simulink model "SimulationLoop_Cpp"  (R2025b)
settings: Solver=VariableStepAuto  StartTime=0.0  StopTime=50  RelTol=1e-3
InitFcn:
  | clear cpp_controller_mex_wrap
values from neighbouring files (symbols this model uses):
  Checkpoints = 0.0 0.0 0.0 0.0 0.0 3.0 0.0 3.0 3.0 3.0 3.0 3.0 3.0 0.0 3.0 0.0 0.0 3.0 0.0 0.0 0.0 0.0 0.0 0.0    [Variables.sldd]
  constantsASTRA = constructConstants    [LoadSimulation.m]    (also in Variables.sldd = 1.275
                0.5
                9.80145
          ; test.m = getEntry(dataSect, 'constantsASTRA'))
  distMode = 1.0    [Variables.sldd]
  dt = 0.005    [Variables.sldd]
  dt_SIM = 0.001    [Variables.sldd]
  HoldTimeReqs = 7.0 5.0 3.0 3.0 3.0 3.0 0.0 0.2    [Variables.sldd]
  IMU_Rate = 1000.0    [Variables.sldd]
  magDistMatrix = 1.0107533427909221 0.036677700291901733 -0.04517693722007296 0.01724346640736241 1.0063753047971795 -0.026153765926105469 -0.0086718404461136721 0.0068524893307729982 1.0715679387945152    [Variables.sldd]
  q = x(7:9)    [TEST1.m]
  u0 = [0; 0; constantsASTRA.g * constantsASTRA.m; 0]    [LoadSimulation.m]    (also in Variables.sldd = 0.0 0.0 12.49684875 0.0)
  x0 = zeros(18,1)    [LoadSimulation.m]    (also in Variables.sldd = 1.0 0.0 0.0 0.0 0.0 0.0 0.0 0.0 0.0 0.0 0.0 0.0 0.0 0.0 0.0 ; run_sim.m = zeros(12,1))
undefined symbols (not defined in the file or in its folder): DiscIntNeverNeededParam, F, Light, MIL
libraries: aerolibnav x2, aerolibwind2 x1, simulink x1
settings Model: PacingRate=5  Creator=antho  LastModifiedBy=pplat
settings OptimizationCC: AccelVerboseBuild=on

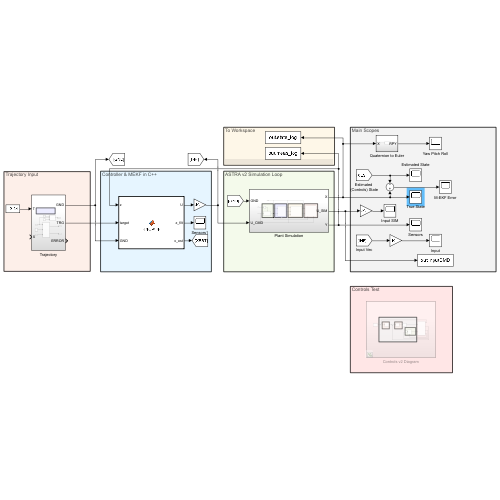
[thumbnail: Simulink's stored preview of the top-level diagram]
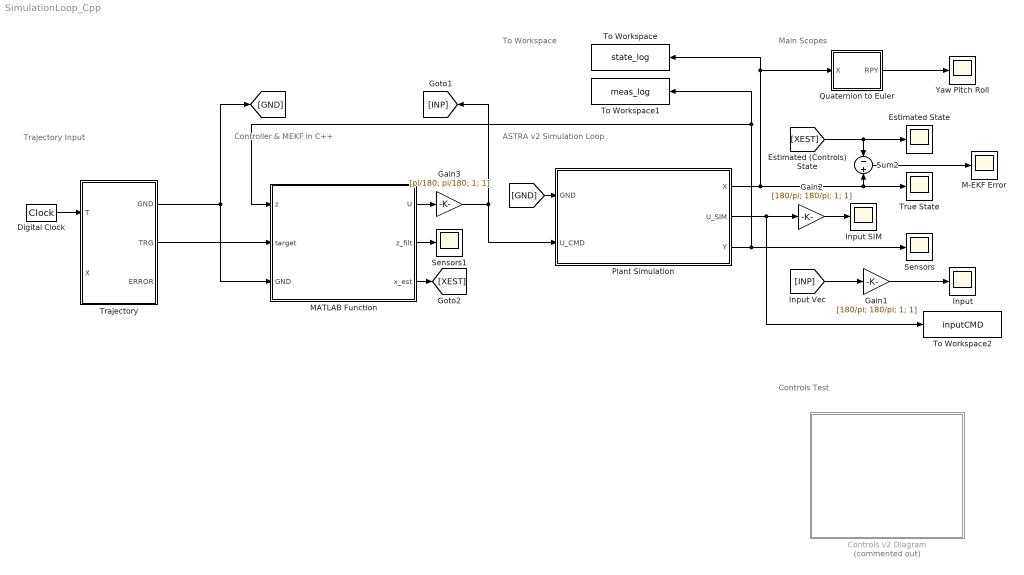
== system SimulationLoop_Cpp ==
  note: To Workspace
  note: Controls Test
  note: Main Scopes
  note: Trajectory Input
  note: Controller & MEKF in C++
  note: ASTRA v2 Simulation Loop
  Controls v2 Diagram : Subsystem  Commented=on
  Digital Clock : DigitalClock  SampleTime=dt_SIM
  Estimated State : Scope
      settings: ActiveDisplayYMinimum=-0.606468253752392  ActiveDisplayYMaximum=3.4359511007845942
  Gain1 : Gain  Gain=[180/pi; 180/pi; 1; 1]
  Gain2 : Gain  Gain=[180/pi; 180/pi; 1; 1]
  Gain3 : Gain  Gain=[pi/180; pi/180; 1; 1]
  Input : Scope
      settings: ActiveDisplayYMinimum=-13.087499976158142  ActiveDisplayYMaximum=17.787499785423279  DataLoggingVariableName=ScopeData6
  Input SIM : Scope
      settings: ActiveDisplayYMinimum=-9.3285969360922252  ActiveDisplayYMaximum=17.369726851522856  DataLoggingVariableName=ScopeData4
  M-EKF Error : Scope
      settings: ActiveDisplayYMinimum=-0.067271632908363993  ActiveDisplayYMaximum=0.0634163897991504  DataLoggingVariableName=ScopeData2
  MATLAB Function : MATLAB Function  TreatAsAtomicUnit=on
  Plant Simulation : Subsystem
  Quaternion to Euler : Subsystem
  Sensors : Scope
      settings: ActiveDisplayYMinimum=-2.5158529896476529  ActiveDisplayYMaximum=2.4618166614919  DataLoggingVariableName=ScopeData3
  Sensors1 : Scope
      settings: ActiveDisplayYMinimum=-5.9307053983211508  ActiveDisplayYMaximum=34.316149324178696  DataLoggingVariableName=ScopeData9
  Sum2 : Sum  Inputs=-|+
  To Workspace : ToWorkspace  VariableName=state_log  SaveFormat=Timeseries  SampleTime=-1
  To Workspace1 : ToWorkspace  VariableName=meas_log  SaveFormat=Timeseries  SampleTime=-1
  To Workspace2 : ToWorkspace  VariableName=inputCMD  SaveFormat=Timeseries  SampleTime=-1
  Trajectory : Subsystem
  True State : Scope
      settings: ActiveDisplayYMinimum=-0.46402431479384865  ActiveDisplayYMaximum=3.346767927011304
  Yaw Pitch Roll : Scope
      settings: ActiveDisplayYMinimum=-2.3625770420783638  ActiveDisplayYMaximum=6.5496164506169734  DataLoggingVariableName=ScopeData7
  wires:
  Digital Clock/1 -> Trajectory/1(T)
  [XEST] -> Sum2/1, Estimated State/1
  Sum2/1 -> M-EKF Error/1
  MATLAB Function/1(U) -> Gain3/1
  Trajectory/1(GND) -> MATLAB Function/3(GND), [GND]
  [INP] -> Gain1/1
  Gain1/1 -> Input/1
  Gain2/1 -> Input SIM/1
  Plant Simulation/2(U_SIM) -> To Workspace2/1, Gain2/1
  Quaternion to Euler/1(RPY) -> Yaw Pitch Roll/1
  [GND] -> Plant Simulation/1(GND)
  Plant Simulation/3(Y) -> To Workspace1/1, MATLAB Function/1(z), Sensors/1
  Plant Simulation/1(X) -> Sum2/2, True State/1, Quaternion to Euler/1(X), To Workspace/1
  Trajectory/2(TRG) -> MATLAB Function/2(target)
  MATLAB Function/2(z_filt) -> Sensors1/1
  MATLAB Function/3(x_est) -> [XEST]
  Gain3/1 -> Plant Simulation/2(U_CMD), [INP]

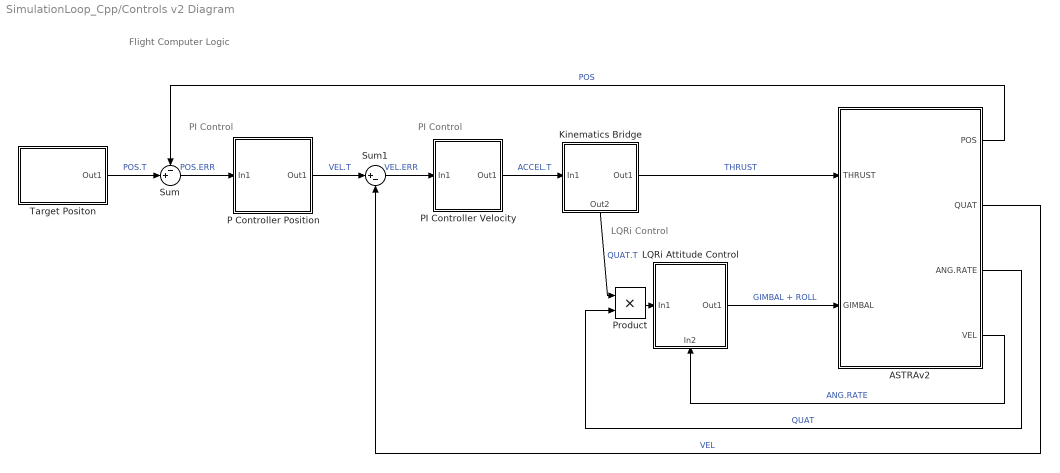
== system SimulationLoop_Cpp/Controls v2 Diagram ==
  note: PI Control
  note: Flight Computer Logic
  note: PI Control
  note: LQRi Control
  ASTRAv2 : Subsystem
  Kinematics Bridge : Subsystem
      settings: PortSchema="{\"entries\":[{\"content\":{\"sides\":[{\"content\":{\"connectorIds\":[\"In1\"]},\"type\":\"ConnectorPlacement.EquallySpacedRectSide\",\"uuid\":\"14f1819f-c5b0-4857-8a3f-059930327852\"},{\"content\":{\"connectorIds\":[\"Out1\"],\"side\":\"RIGHT\"},\"type\":\"ConnectorPlacement.EquallySpacedRectSide\",\"uuid\":\"f1c93ae3-8d17-4b74-967d-9d6328e115fb\"},{\"content\":{\"side\":\"TOP\"},\"type\":\"ConnectorPlacement.EquallySpacedRectSide\",\"uuid\":\"bc82f49d-1f27-4136-b175-63a6ad0dbf5b\"},{\"content\":{\"connectorIds\":[\"Out2\"],\"side\":\"BOTTOM\"},\"type\":\"ConnectorPlacement.EquallySpacedRectSide\",\"uuid\":\"6dcf9527-a6d9-4dea-a2bb-d98c67e6f046\"}]},\"type\":\"ConnectorPlacement.EquallySpacedConnector\",\"uuid\":\"f166f20b-cbf6-467f-83b3-19efe4727134\"}],\"packageUris\":[\"http://schema.mathworks.com/mf0/Connector/R2020b\"],\"version\":\"1.0\"}"
  LQRi Attitude Control : Subsystem
      settings: PortSchema="{\"entries\":[{\"content\":{\"sides\":[{\"content\":{\"connectorIds\":[\"In1\"]},\"type\":\"ConnectorPlacement.EquallySpacedRectSide\",\"uuid\":\"cd9cee5f-4e02-4c25-b158-b6d381dcbc8d\"},{\"content\":{\"connectorIds\":[\"Out1\"],\"side\":\"RIGHT\"},\"type\":\"ConnectorPlacement.EquallySpacedRectSide\",\"uuid\":\"2ef087dd-7fcc-4555-b2da-05ccf598bd0a\"},{\"content\":{\"side\":\"TOP\"},\"type\":\"ConnectorPlacement.EquallySpacedRectSide\",\"uuid\":\"5427ed8c-500e-4860-8e5f-93d13574dd24\"},{\"content\":{\"connectorIds\":[\"In2\"],\"side\":\"BOTTOM\"},\"type\":\"ConnectorPlacement.EquallySpacedRectSide\",\"uuid\":\"f48b80df-9658-4fd9-b967-6adbaff8a875\"}]},\"type\":\"ConnectorPlacement.EquallySpacedConnector\",\"uuid\":\"547d8ec4-1c4e-4f3b-85b8-72bd650a229d\"}],\"packageUris\":[\"http://schema.mathworks.com/mf0/Connector/R2020b\"],\"version\":\"1.0\"}"
  P Controller Position : Subsystem
  PI Controller Velocity : Subsystem
  Product : Product
  Sum : Sum  Inputs=-+|
  Sum1 : Sum  Inputs=|+-
  Target Positon : Subsystem
  wires:
  P Controller Position/1(Out1) -> Sum1/1  "VEL.T"
  Sum1/1 -> PI Controller Velocity/1(In1)  "VEL.ERR"
  PI Controller Velocity/1(Out1) -> Kinematics Bridge/1(In1)  "ACCEL.T"
  Sum/1 -> P Controller Position/1(In1)  "POS.ERR"
  Kinematics Bridge/2(Out2) -> Product/1  "QUAT.T"
  Product/1 -> LQRi Attitude Control/1(In1)
  LQRi Attitude Control/1(Out1) -> ASTRAv2/2("GIMBAL ")  "GIMBAL + ROLL"
  Kinematics Bridge/1(Out1) -> ASTRAv2/1(THRUST)  "THRUST"
  Target Positon/1(Out1) -> Sum/2  "POS.T"
  ASTRAv2/1(POS) -> Sum/1  "POS"
  ASTRAv2/2(QUAT) -> Sum1/2  "VEL"
  ASTRAv2/3(ANG.RATE) -> Product/2  "QUAT"
  ASTRAv2/4(VEL) -> LQRi Attitude Control/2(In2)  "ANG.RATE"

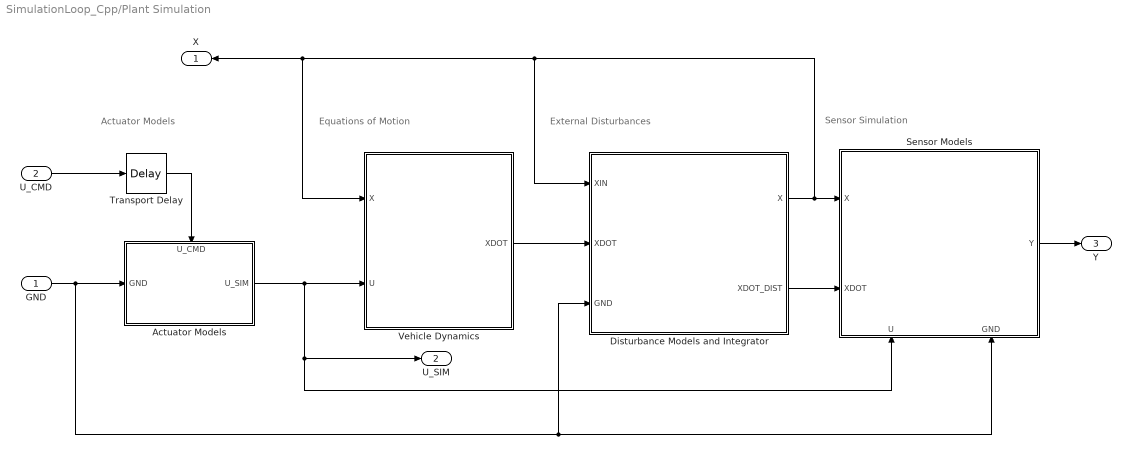
== system SimulationLoop_Cpp/Plant Simulation ==
  note: Equations of Motion
  note: Actuator Models
  note: External Disturbances
  note: Sensor Simulation
  GND : Inport
  U_CMD : Inport  Port=2
  Actuator Models : Subsystem
      settings: PortSchema="{\"entries\":[{\"content\":{\"sides\":[{\"content\":{\"connectorIds\":[\"In1\"]},\"type\":\"ConnectorPlacement.EquallySpacedRectSide\",\"uuid\":\"54343072-6023-41e9-a0f6-81f6bed17e05\"},{\"content\":{\"connectorIds\":[\"Out1\"],\"side\":\"RIGHT\"},\"type\":\"ConnectorPlacement.EquallySpacedRectSide\",\"uuid\":\"2ed3290f-d38b-41d8-95ae-d88068502334\"},{\"content\":{\"connectorIds\":[\"In2\"],\"side\":\"TOP\"},\"type\":\"ConnectorPlacement.EquallySpacedRectSide\",\"uuid\":\"e9e41c57-b871-4be2-92e8-dfbbf995d6b0\"}]},\"type\":\"ConnectorPlacement.EquallySpacedConnector\",\"uuid\":\"c037521e-b20b-40c6-bb74-3aafe8fc1476\"}],\"packageUris\":[\"http://schema.mathworks.com/mf0/Connector/R2020b\"],\"version\":\"1.0\"}"
  Disturbance Models and Integrator : Subsystem
  Sensor Models : Subsystem
      settings: PortSchema="{\"entries\":[{\"content\":{\"sides\":[{\"content\":{\"connectorIds\":[\"In1\",\"In2\"]},\"type\":\"ConnectorPlacement.EquallySpacedRectSide\",\"uuid\":\"9bc4a206-bba4-4c50-88a9-89b0392ab722\"},{\"content\":{\"connectorIds\":[\"Out1\"],\"side\":\"RIGHT\"},\"type\":\"ConnectorPlacement.EquallySpacedRectSide\",\"uuid\":\"162bbd17-e1b8-4f29-9191-53e17e38d79d\"},{\"content\":{\"side\":\"TOP\"},\"type\":\"ConnectorPlacement.EquallySpacedRectSide\",\"uuid\":\"c56a23db-6a5c-435f-99fd-d50fc9dbdc94\"},{\"content\":{\"connectorIds\":[\"In3\",\"In4\"],\"side\":\"BOTTOM\"},\"type\":\"ConnectorPlacement.EquallySpacedRectSide\",\"uuid\":\"e0c2a0dc-3b7a-40ac-8345-28e7bf7b9405\"}]},\"type\":\"ConnectorPlacement.EquallySpacedConnector\",\"uuid\":\"d1c29f55-9be5-4f45-9d70-06beba2c2f44\"}],\"packageUris\":[\"http://schema.mathworks.com/mf0/Connector/R2020b\"],\"version\":\"1.0\"}"
  Transport Delay : TransportDelay  DelayTime=0.02  InitialOutput=u0
  Vehicle Dynamics : Subsystem
  X : Outport
  U_SIM : Outport  Port=2
  Y : Outport  Port=3
  wires:
  Vehicle Dynamics/1(XDOT) -> Disturbance Models and Integrator/2(XDOT)
  Sensor Models/1(Y) -> Y/1
  GND/1 -> Actuator Models/1(GND), Sensor Models/4(GND), Disturbance Models and Integrator/3(GND)
  Disturbance Models and Integrator/1(X) -> Disturbance Models and Integrator/1(XIN), Vehicle Dynamics/1(X), X/1, Sensor Models/1(X)
  Disturbance Models and Integrator/2(XDOT_DIST) -> Sensor Models/2(XDOT)
  Actuator Models/1(U_SIM) -> U_SIM/1, Sensor Models/3(U), Vehicle Dynamics/2(U)
  U_CMD/1 -> Transport Delay/1
  Transport Delay/1 -> Actuator Models/2(U_CMD)

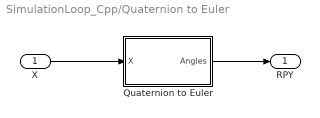
== system SimulationLoop_Cpp/Quaternion to Euler ==
  X : Inport
  Quaternion to Euler : MATLAB Function  TreatAsAtomicUnit=on
  RPY : Outport
  wires:
  X/1 -> Quaternion to Euler/1(X)
  Quaternion to Euler/1(Angles) -> RPY/1

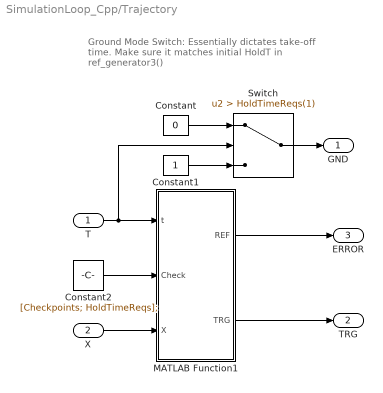
== system SimulationLoop_Cpp/Trajectory ==
  note: Ground Mode Switch:
      | Essentially dictates take-off time.
      | Make sure it matches initial HoldT
      | in ref_generator3()
  T : Inport
  X : Inport  Port=2
  Constant : Constant  Value=0
  Constant1 : Constant
  Constant2 : Constant  Value=[Checkpoints; HoldTimeReqs];
  MATLAB Function1 : MATLAB Function  TreatAsAtomicUnit=on
  Switch : Switch  Criteria=u2 > Threshold  Threshold=HoldTimeReqs(1)  SaturateOnIntegerOverflow=off  InputSameDT=off
  GND : Outport
  TRG : Outport  Port=2
  ERROR : Outport  Port=3
  wires:
  T/1 -> Switch/2, MATLAB Function1/1(t)
  X/1 -> MATLAB Function1/3(X)
  MATLAB Function1/1(REF) -> ERROR/1
  Constant/1 -> Switch/1
  Constant1/1 -> Switch/3
  Switch/1 -> GND/1
  Constant2/1 -> MATLAB Function1/2(Check)
  MATLAB Function1/2(TRG) -> TRG/1

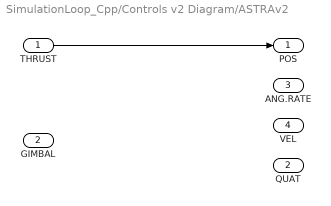
== system SimulationLoop_Cpp/Controls v2 Diagram/ASTRAv2 ==
  THRUST : Inport
  "GIMBAL " : Inport  Port=2
  POS : Outport
  QUAT : Outport  Port=2
  ANG.RATE : Outport  Port=3
  VEL : Outport  Port=4
  wires:
  THRUST/1 -> POS/1

== system SimulationLoop_Cpp/Controls v2 Diagram/Kinematics Bridge ==
  In1 : Inport
  Out1 : Outport
  Out2 : Outport  Port=2
  wires:
  In1/1 -> Out2/1, Out1/1

== system SimulationLoop_Cpp/Controls v2 Diagram/LQRi Attitude Control ==
  In1 : Inport
  In2 : Inport  Port=2
  Out1 : Outport
  wires:
  In1/1 -> Out1/1

== system SimulationLoop_Cpp/Controls v2 Diagram/P Controller Position ==
  In1 : Inport
  Out1 : Outport
  wires:
  In1/1 -> Out1/1

== system SimulationLoop_Cpp/Controls v2 Diagram/PI Controller Velocity ==
  In1 : Inport
  Out1 : Outport
  wires:
  In1/1 -> Out1/1

== system SimulationLoop_Cpp/Controls v2 Diagram/Target Positon ==
  Out1 : Outport
  wires:
  ? -> Out1/1

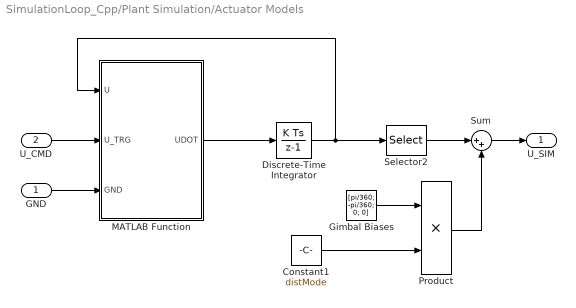
== system SimulationLoop_Cpp/Plant Simulation/Actuator Models ==
  GND : Inport
  U_CMD : Inport  Port=2
  Constant1 : Constant  Value=distMode
  Discrete-Time Integrator : DiscreteIntegrator  InitialCondition=[zeros(4,1); u0(3); 0]  SampleTime=-1  ICPrevOutput=DiscIntNeverNeededParam  ICPrevScaledInput=DiscIntNeverNeededParam
  Gimbal Biases : Constant  Value=[pi/360; -pi/360; 0; 0]
  MATLAB Function : MATLAB Function  TreatAsAtomicUnit=on
  Product : Product
  Selector2 : Selector  InputPortWidth=6  IndexOptions=Index vector (dialog)  Indices=[1 3 5 6]  OutputSizes=1
  Sum : Sum  Inputs=|++
  U_SIM : Outport
  wires:
  U_CMD/1 -> MATLAB Function/2(U_TRG)
  MATLAB Function/1(UDOT) -> Discrete-Time Integrator/1
  Discrete-Time Integrator/1 -> MATLAB Function/1(U), Selector2/1
  GND/1 -> MATLAB Function/3(GND)
  Sum/1 -> U_SIM/1
  Selector2/1 -> Sum/1
  Gimbal Biases/1 -> Product/1
  Product/1 -> Sum/2
  Constant1/1 -> Product/2

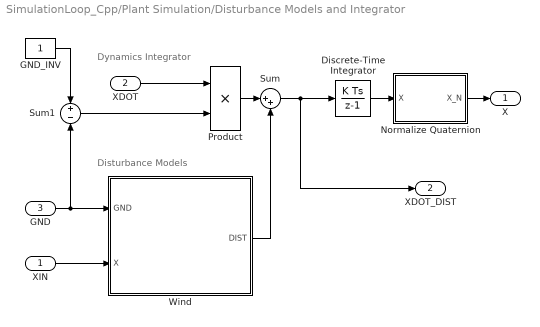
== system SimulationLoop_Cpp/Plant Simulation/Disturbance Models and Integrator ==
  note: Disturbance Models
  note: Dynamics Integrator
  XIN : Inport
  XDOT : Inport  Port=2
  GND : Inport  Port=3
  Discrete-Time Integrator : DiscreteIntegrator  InitialCondition=x0  SampleTime=-1  ICPrevOutput=DiscIntNeverNeededParam  ICPrevScaledInput=DiscIntNeverNeededParam
  GND_INV : Constant
  Normalize Quaternion : MATLAB Function  TreatAsAtomicUnit=on
  Product : Product
  Sum : Sum  Inputs=|++
  Sum1 : Sum  Inputs=+|-
  Wind : Subsystem
  X : Outport
  XDOT_DIST : Outport  Port=2
  wires:
  Discrete-Time Integrator/1 -> Normalize Quaternion/1(X)
  XIN/1 -> Wind/2(X)
  Wind/1(DIST) -> Sum/2
  XDOT/1 -> Product/1
  GND_INV/1 -> Sum1/1
  Sum1/1 -> Product/2
  GND/1 -> Wind/1(GND), Sum1/2
  Product/1 -> Sum/1
  Sum/1 -> Discrete-Time Integrator/1, XDOT_DIST/1
  Normalize Quaternion/1(X_N) -> X/1

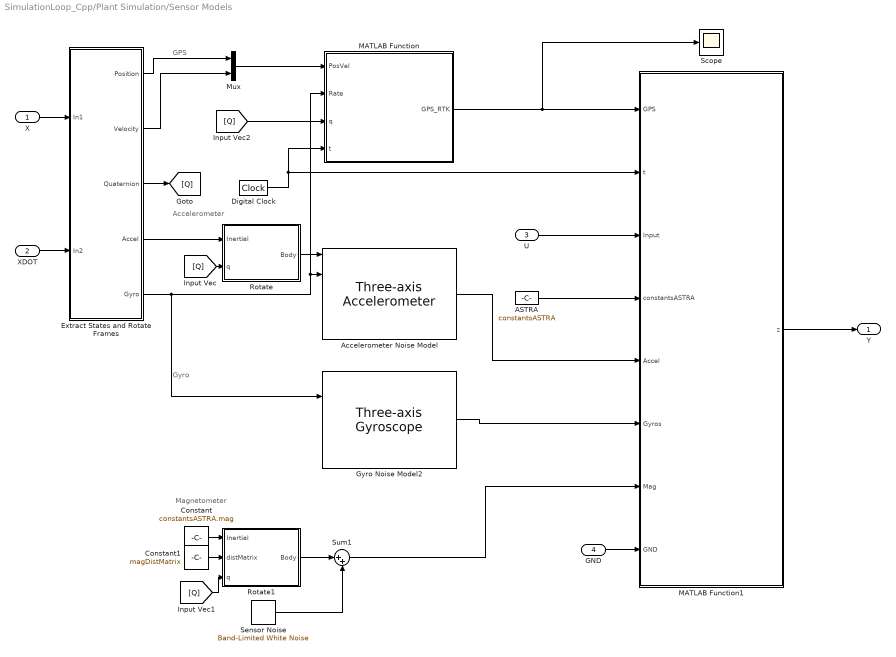
== system SimulationLoop_Cpp/Plant Simulation/Sensor Models ==
  note: Gyro
  note: Accelerometer
  note: Magnetometer
  note: GPS
  X : Inport
  XDOT : Inport  Port=2
  U : Inport  Port=3
  GND : Inport  Port=4
  ASTRA : Constant  Value=constantsASTRA  OutDataTypeStr=Bus: slBus1
  Accelerometer Noise Model : aerolibnav/Three-axis Accelerometer  units=Metric (MKS)  acc=[0 0 0.15]  gtype=on  dtype_a=on  w_a=190  z_a=0.707  a_sf_cc=eye(3)  a_bias=accelBias  a_Ts=1 / IMU_Rate  a_rand=on  a_seeds=[23093 23094 23095]  a_pow=ones(1,3) * 0.008^2 * 1 / IMU_Rate  a_sat="[-inf  -inf  -inf  inf inf inf]"
  Constant : Constant  Value=constantsASTRA.mag
  Constant1 : Constant  Value=magDistMatrix
  Digital Clock : DigitalClock  SampleTime=dt_SIM
  Extract States and Rotate Frames : Subsystem
  Gyro Noise Model2 : aerolibnav/Three-axis Gyroscope  dtype_g=on  w_g=190  z_g=0.707  g_sf_cc=eye(3)  g_bias=gyroBias  g_sen=0  g_Ts=1 / IMU_Rate  g_rand=on  g_seeds=[23093 23094 23095]  g_pow=ones(1,3) * 0.003^2 * dt  g_sat="[-inf  -inf  -inf  inf inf inf]"
  MATLAB Function : MATLAB Function  TreatAsAtomicUnit=on
  MATLAB Function1 : MATLAB Function  TreatAsAtomicUnit=on
  Mux : Mux  Inputs=2
  Rotate : MATLAB Function  TreatAsAtomicUnit=on
  Rotate1 : MATLAB Function  TreatAsAtomicUnit=on
  Scope : Scope
      settings: ActiveDisplayYMinimum=-1  ActiveDisplayYMaximum=1  DataLoggingVariableName=ScopeData10
  Sensor Noise : simulink/Sources/Band-Limited White Noise  Cov=(4E-4)^2  Ts=dt_SIM  seed=[23341,23342,23343]
  Sum1 : Sum  Inputs=|++
  Y : Outport
  wires:
  X/1 -> Extract States and Rotate Frames/1(In1)
  XDOT/1 -> Extract States and Rotate Frames/2(In2)
  Digital Clock/1 -> MATLAB Function/4(t), MATLAB Function1/2(t)
  Extract States and Rotate Frames/5(Gyro) -> Accelerometer Noise Model/2, MATLAB Function/2(Rate), Gyro Noise Model2/1
  Extract States and Rotate Frames/3(Quaternion) -> [Q]
  Rotate/1(Body) -> Accelerometer Noise Model/1
  Extract States and Rotate Frames/4(Accel) -> Rotate/1(Inertial)
  [Q] -> Rotate/2(q)
  Constant/1 -> Rotate1/1(Inertial)
  [Q] -> Rotate1/3(q)
  Sensor Noise/1 -> Sum1/2
  Rotate1/1(Body) -> Sum1/1
  Sum1/1 -> MATLAB Function1/7(Mag)
  MATLAB Function/1(GPS_RTK) -> Scope/1, MATLAB Function1/1(GPS)
  Accelerometer Noise Model/1 -> MATLAB Function1/5(Accel)
  Gyro Noise Model2/1 -> MATLAB Function1/6(Gyros)
  MATLAB Function1/1(z) -> Y/1
  ASTRA/1 -> MATLAB Function1/4(constantsASTRA)
  Extract States and Rotate Frames/2(Velocity) -> Mux/2
  Mux/1 -> MATLAB Function/1(PosVel)
  Extract States and Rotate Frames/1(Position) -> Mux/1
  U/1 -> MATLAB Function1/3(Input)
  GND/1 -> MATLAB Function1/8(GND)
  Constant1/1 -> Rotate1/2(distMatrix)
  [Q] -> MATLAB Function/3(q)

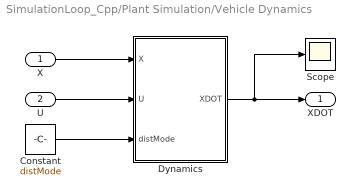
== system SimulationLoop_Cpp/Plant Simulation/Vehicle Dynamics ==
  X : Inport
  U : Inport  Port=2
  Constant : Constant  Value=distMode
  Dynamics : MATLAB Function  TreatAsAtomicUnit=on
  Scope : Scope
      settings: ActiveDisplayYMinimum=-0.093144832224715035  ActiveDisplayYMaximum=0.26958232579352592  DataLoggingVariableName=ScopeData11
  XDOT : Outport
  wires:
  Dynamics/1(XDOT) -> Scope/1, XDOT/1
  U/1 -> Dynamics/2(U)
  X/1 -> Dynamics/1(X)
  Constant/1 -> Dynamics/3(distMode)

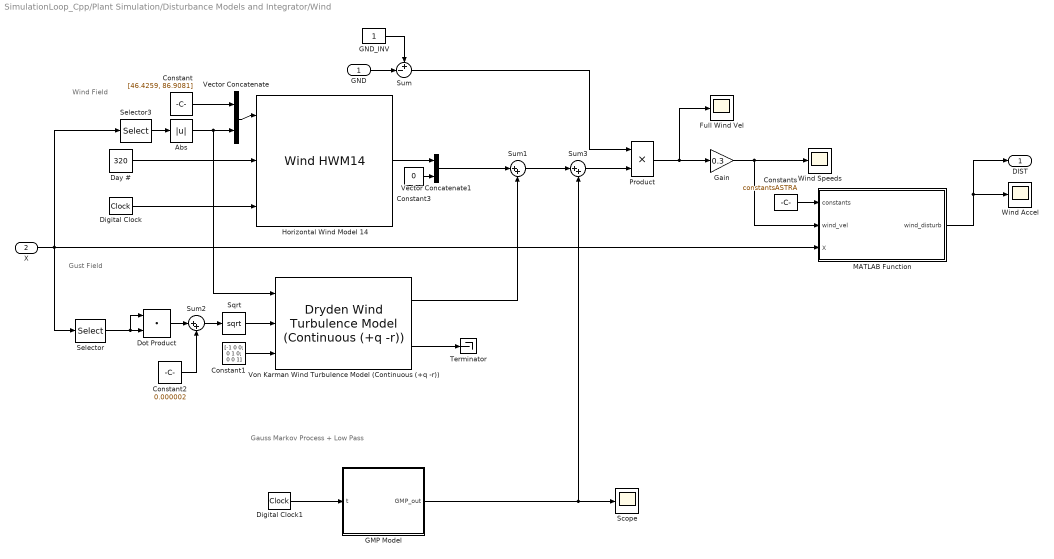
== system SimulationLoop_Cpp/Plant Simulation/Disturbance Models and Integrator/Wind ==
  note: Gauss Markov Process + Low Pass
  note: Gust Field
  note: Wind Field
  GND : Inport
  X : Inport  Port=2
  Abs : Abs  SaturateOnIntegerOverflow=off
  Constant : Constant  Value=[46.4259, 86.9081]
  Constant1 : Constant  Value=[-1 0 0; 0 1 0; 0 0 1]
  Constant2 : Constant  Value=0.000002
  Constant3 : Constant  Value=0
  Constants : Constant  Value=constantsASTRA  OutDataTypeStr=Bus: slBus1
  Day # : Constant  Value=320
  Digital Clock : DigitalClock  SampleTime=dt_SIM
  Digital Clock1 : DigitalClock  SampleTime=dt_SIM
  Dot Product : DotProduct  OutDataTypeStr=Inherit: Inherit via internal rule
  Full Wind Vel : Scope
      settings: ActiveDisplayYMinimum=-5.9330847029288414  ActiveDisplayYMaximum=4.4700897462030218  DataLoggingVariableName=ScopeData13
  GMP Model : MATLAB Function  TreatAsAtomicUnit=on
  GND_INV : Constant
  Gain : Gain  Gain=0.3
  Horizontal Wind Model 14 : WindHWM14
  MATLAB Function : MATLAB Function  TreatAsAtomicUnit=on
  Product : Product
  Scope : Scope
      settings: ActiveDisplayYMinimum=-2.8676060433464485  ActiveDisplayYMaximum=2.8612107779538238  DataLoggingVariableName=ScopeData14
  Selector : Selector  InputPortWidth=16  IndexOptions=Index vector (dialog)  Indices=[8:10]  OutputSizes=1
  Selector3 : Selector  InputPortWidth=16  IndexOptions=Index vector (dialog)  Indices=7  OutputSizes=1
  Sqrt : Sqrt
  Sum : Sum  Inputs=+-|
  Sum1 : Sum  Inputs=|++
  Sum2 : Sum  Inputs=|++
  Sum3 : Sum  Inputs=|++
  Terminator : Terminator
  Vector Concatenate : Concatenate
  Vector Concatenate1 : Concatenate
  Von Karman Wind Turbulence Model (Continuous (+q -r)) : aerolibwind2/Dryden Wind Turbulence Model  (Continuous (+q -r))  units=Metric (MKS)  spec=MIL-F-8785C  model=Continuous Von Karman (+q -r)  W20=15  Wdeg=0  TurbProb=10^-2 - Light  L_high=762  Wingspan=10  ts=0.1  Seed=[23341 23342 23343 23344]  T_on=on
      settings: LibrarySourceBlock=|
      | aerolibwind2/Von Karman Wind Turbulence Model
      | (Continuous (+q -r))
  Wind Accel : Scope
      settings: ActiveDisplayYMinimum=-0.93847040858698449  ActiveDisplayYMaximum=0.85102417935944119  DataLoggingVariableName=ScopeData5
  Wind Speeds : Scope
      settings: ActiveDisplayYMinimum=-6.0032131159962416  ActiveDisplayYMaximum=4.44789373969359  DataLoggingVariableName=ScopeData5
  DIST : Outport
  wires:
  Digital Clock/1 -> Horizontal Wind Model 14/3
  Day #/1 -> Horizontal Wind Model 14/2
  MATLAB Function/1(wind_disturb) -> DIST/1, Wind Accel/1
  Vector Concatenate/1 -> Horizontal Wind Model 14/1
  Selector3/1 -> Abs/1
  Constant/1 -> Vector Concatenate/1
  GND/1 -> Sum/2
  Sum/1 -> Product/1
  GND_INV/1 -> Sum/1
  Horizontal Wind Model 14/1 -> Vector Concatenate1/1
  Constants/1 -> MATLAB Function/1(constants)
  Selector/1 -> Dot Product/1, Dot Product/2
  Sqrt/1 -> Von Karman Wind Turbulence Model (Continuous (+q -r))/2
  Von Karman Wind Turbulence Model (Continuous (+q -r))/1 -> Sum1/2
  Constant1/1 -> Von Karman Wind Turbulence Model (Continuous (+q -r))/3
  Sum2/1 -> Sqrt/1
  Dot Product/1 -> Sum2/1
  Constant2/1 -> Sum2/2
  X/1 -> Selector3/1, MATLAB Function/3(X), Selector/1
  Abs/1 -> Vector Concatenate/2, Von Karman Wind Turbulence Model (Continuous (+q -r))/1
  Product/1 -> Full Wind Vel/1, Gain/1
  Vector Concatenate1/1 -> Sum1/1
  Constant3/1 -> Vector Concatenate1/2
  Von Karman Wind Turbulence Model (Continuous (+q -r))/2 -> Terminator/1
  Gain/1 -> Wind Speeds/1, MATLAB Function/2(wind_vel)
  Sum3/1 -> Product/2
  Sum1/1 -> Sum3/1
  GMP Model/1(GMP_out) -> Scope/1, Sum3/2
  Digital Clock1/1 -> GMP Model/1(t)

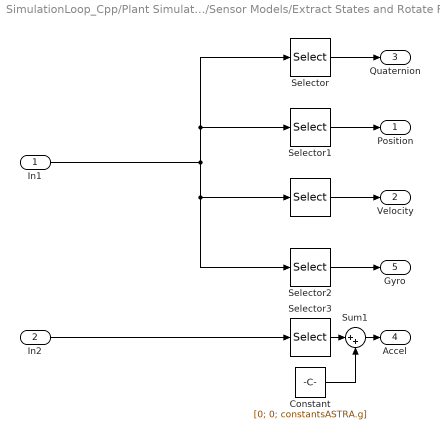
== system SimulationLoop_Cpp/Plant Simulation/Sensor Models/Extract States and Rotate Frames ==
  In1 : Inport
  In2 : Inport  Port=2
  "  " : Selector  InputPortWidth=16  IndexOptions=Index vector (dialog)  Indices=[8:10]  OutputSizes=1
  Constant : Constant  Value=[0; 0; constantsASTRA.g]
  Selector : Selector  InputPortWidth=16  IndexOptions=Index vector (dialog)  Indices=[1:4]  OutputSizes=1
  Selector1 : Selector  InputPortWidth=16  IndexOptions=Index vector (dialog)  Indices=[5:7]  OutputSizes=1
  Selector2 : Selector  InputPortWidth=16  IndexOptions=Index vector (dialog)  Indices=[11:13]  OutputSizes=1
  Selector3 : Selector  InputPortWidth=16  IndexOptions=Index vector (dialog)  Indices=[8:10]  OutputSizes=1
  Sum1 : Sum  Inputs=|++
  Position : Outport
  Velocity : Outport  Port=2
  Quaternion : Outport  Port=3
  Accel : Outport  Port=4
  Gyro : Outport  Port=5
  wires:
  Selector/1 -> Quaternion/1
  Selector1/1 -> Position/1
  "  "/1 -> Velocity/1
  Selector2/1 -> Gyro/1
  Selector3/1 -> Sum1/1
  Sum1/1 -> Accel/1
  Constant/1 -> Sum1/2
  In1/1 -> Selector1/1, Selector/1, Selector2/1, "  "/1
  In2/1 -> Selector3/1

== matlab function SimulationLoop_Cpp/Plant Simulation/Sensor Models/MATLAB Function1 ==
  data: GPS input; t input; Input input; constantsASTRA input; Accel input; z output; Gyros input; Mag input; GND input
function z = SensorFrequency(GPS, t, Input, constantsASTRA, Accel, Gyros, Mag, GND)
%% Add Thrust Varying Oscillation
persistent phase lastT
if isempty(phase)
    phase = 0;
    lastT = 0;
end
dt = t - lastT;
lastT = t;

% Thrust vibration generator
Track = [1.3525    42.6278];
THRUST = Input(3) / constantsASTRA.MaxT * 100;
w = 2 * pi * (Track(1) * THRUST + Track(2) + 1 * randn());
phase = phase + w * dt;
MaxAmplAccel = 7;
MaxAmplGyro = 0.2;
Accel = Accel + MaxAmplAccel * THRUST / 100 * sin(phase) * (1 - GND);
Gyros = Gyros + MaxAmplGyro * THRUST / 100 * sin(phase) * (1 - GND);
z = [Accel; Gyros; Mag; GPS];

== matlab function SimulationLoop_Cpp/Plant Simulation/Disturbance Models and Integrator/Wind/GMP Model ==
  data: t input; GMP_out output
function GMP_out = GMP(t)

persistent errorval lastTime EMA
if isempty(errorval)
    errorval = 0;
    EMA = 0;
    lastTime = 0;  % Update last timestamp
end

dT = t - lastTime;

% First order Gauss Markov Process for additional disturbance
decay = 10;
beta = exp(-dT / decay);
covar = 1;
errorval = beta * errorval + sqrt(1 - beta^2) * covar * randn;

% EMA Step to kill High Freq. Noise
EMA = ExpMovingAvg(errorval, EMA, 0.05);
GMP_out = EMA * ones(3,1);
lastTime = t;

== matlab function SimulationLoop_Cpp/Plant Simulation/Vehicle Dynamics/Dynamics ==
  data: X input; XDOT output; U input; distMode input
function XDOT = Dynamics(X, U, distMode)
if distMode == 1
    XDOT = disturbedDynamics(X, U);
else
    XDOT = nominalDynamics(X, U);
end
if X(7) < 0
    XDOT(10) = XDOT(10) + max(-1000* X(7) - 200 * X(10), 0);
end

== matlab function SimulationLoop_Cpp/Trajectory/MATLAB Function1 ==
  data: t input; Check input; X input; REF output; TRG output
function [REF, TRG] = RefSignal(t, Check, X)

Checkpoints = Check(1:3, :);
HoldReqs = Check(4, :);
[REF, TRG] = ref_generator3(X, t, Checkpoints, HoldReqs);

== matlab function SimulationLoop_Cpp/Plant Simulation/Sensor Models/Rotate ==
  data: Inertial input; Body output; q input
function Body = Rotate(Inertial, q)
Body = quatRot(q) * Inertial;

== matlab function SimulationLoop_Cpp/Plant Simulation/Disturbance Models and Integrator/Wind/MATLAB Function ==
  data: constants input; wind_vel input; X input; wind_disturb output
function wind_disturb = wind_sim(constants, wind_vel, X)

wind_disturb = wind(constants, wind_vel, X);

== matlab function SimulationLoop_Cpp/Plant Simulation/Actuator Models/MATLAB Function ==
  data: U input; UDOT output; U_TRG input; GND input
function UDOT = Actuators(U, U_TRG, GND)

    UDOT = ActuatorDynamics(U, U_TRG, GND);
end

== matlab function SimulationLoop_Cpp/Quaternion to Euler/Quaternion to Euler ==
  data: X input; Angles output
function Angles = q2eul(X)

% Complete quaternion
q = X(1:4);

% Quaternion to Euler Angles
Roll = atan2(2*(q(1) * q(2) + q(3) * q(4)), 1 - 2*(q(2)^2 + q(3)^2));
Pitch = asin(2*(q(1) * q(3) - q(4) * q(2)));
Yaw = atan2(2*(q(1) * q(4) + q(2) * q(3)), 1 - 2*(q(3)^2 + q(4)^2));

% Angle Vector
Angles = [Roll; Pitch; Yaw] * 180/pi;

== matlab function SimulationLoop_Cpp/MATLAB Function ==
  data: z input; U output; target input; GND input; z_filt output; x_est output
function [U, z_filt, x_est] = cpp_wrap(z, target, GND)
    coder.extrinsic('cpp_controller_mex_wrap');
    U = zeros(4,1);   % must predefine size/type
    z_filt = zeros(15, 1);
    x_est = zeros(13, 1);
    [U, z_filt, x_est] = cpp_controller_mex_wrap(z, target, GND, 1/1000);

== matlab function SimulationLoop_Cpp/Plant Simulation/Disturbance Models and Integrator/Normalize Quaternion ==
  data: X input; X_N output
function X_N = fcn(X)
X_N = [X(1:4) / norm(X(1:4)); X(5:end)];

== matlab function SimulationLoop_Cpp/Plant Simulation/Sensor Models/Rotate1 ==
  data: Inertial input; distMatrix input; Body output; q input
function Body = Rotate(Inertial, distMatrix, q)
Body = quatRot(q) * (distMatrix * Inertial + 0.05 * ones(3,1));

== matlab function SimulationLoop_Cpp/Plant Simulation/Sensor Models/MATLAB Function ==
  data: PosVel input; Rate input; q input; GPS_RTK output; t input
function GPS_RTK = GPS(PosVel, Rate, q, t)

R_b2i = quatRot(q)';
GPS_RTK = GPS_Sim(PosVel, Rate, R_b2i, t);
